simulink model "cube_2d_simulation_model"  (R2015b)
settings: Solver=FixedStepAuto  StartTime=0.0  StopTime=10  FixedStep=T_onboard  RelTol=1e-3
PreLoadFcn:
  | cubeinit
InitFcn:
  | cubeparameters
values from neighbouring files (symbols this model uses):
  a_max = 2*g    [cubeparameters.m]
  a_scaling = 16384    [cubeparameters.m]
  cub_friction = 0.0001    [Linearized_system.m]
  cube_start_angle = 0.1*deg_    (= 0.00174532925199)    [cubeparameters.m]
  deg_ = pi/180    (= 0.0174532925199)    [cubeparameters.m]    (also in testa.m)
  Fcube = 0.0001    [Linearized_system.m]
  Fwheel = 0.05*10^-3    (= 5e-05)    [Linearized_system.m]
  g = 9.81    [CalculateImuErrors2D.m]    (also in Linearized_system.m; plotimudata.m; run_simulation_2D.m)
  I_cube = 2*(I_p + m_s*2*(s/2)^2)      + 2*(I_o + m_s*s^2/4)      + 2*(I_o + m_s*((s/2)^2+s^2))    (= 0.0610225)    [cubeparameters.m]
  I_motor = 1.81*10^-5    (= 1.81e-05)    [Linearized_system.m]
  I_total = 0.035    [Linearized_system.m]
  I_wheel = 8*10^-4    (= 0.0008)    [Linearized_system.m]    (also in cubeparameters.m = 0.000796068)
  imu_intended_alignment = [0;0;-135*deg_]    [cubeparameters.m]
  imu_misalignment = [0;0;0]*deg_    [cubeparameters.m]
  Km_alt = 5.115537e-3    (= 0.005115537)    [cubeparameters.m]
  Kt = 38*10^-3    (= 0.038)    [Linearized_system.m]
  Kv = 36.9*10^-3    (= 0.0369)    [Linearized_system.m]
  L = 0.463*10^-3    (= 0.000463)    [Linearized_system.m]
  l_corner2cog = side_length/sqrt(2)    [cubeparameters.m]
  Lcub = sqrt((mass_centrum_oneside^2)*2) -0.085    [Linearized_system.m]
  Load = 6*10^-4    (= 0.0006)    [Linearized_system.m]
  Lwheel = sqrt((0.1^2)*2) -0.1    [Linearized_system.m]
  mass_cube = 3.487*kg_    (= 3.487)    [cubeparameters.m]    (also in theoreticalmomentofinertia.m)
  maxvinkel = pi/4    (= 0.785398163397)    [Linearized_system.m]
  Mcub = 2.083-Mwheel    (= 1.81)    [Linearized_system.m]
  Mwheel = 0.273    [Linearized_system.m]
  R = 0.608    [Linearized_system.m]    (also in OrientationView.m = (eye(3) - 0.9*A(:, 3)*A(:, 3)'/(A(:, 3)'*A(:, 3))))
  r_cube2imu = e2t([0;0;pi/4])*[55;70;10]*mm_    [cubeparameters.m]
  sensor_seed = 123123    [cubeparameters.m]
  T_onboard = 0.002*s_    (= 0.002)    [cubeparameters.m]
  w_max = 250*deg_/s_    (= 4.36332312999)    [cubeparameters.m]
  w_scaling = 131    [cubeparameters.m]
  wheel_friction = 0.05*10^-3    (= 5e-05)    [Linearized_system.m]
libraries: cube_lib x10, simulink x5, stm32f4_io_lib x2
settings Model: Creator=Stefan  LastModifiedBy=Stefan

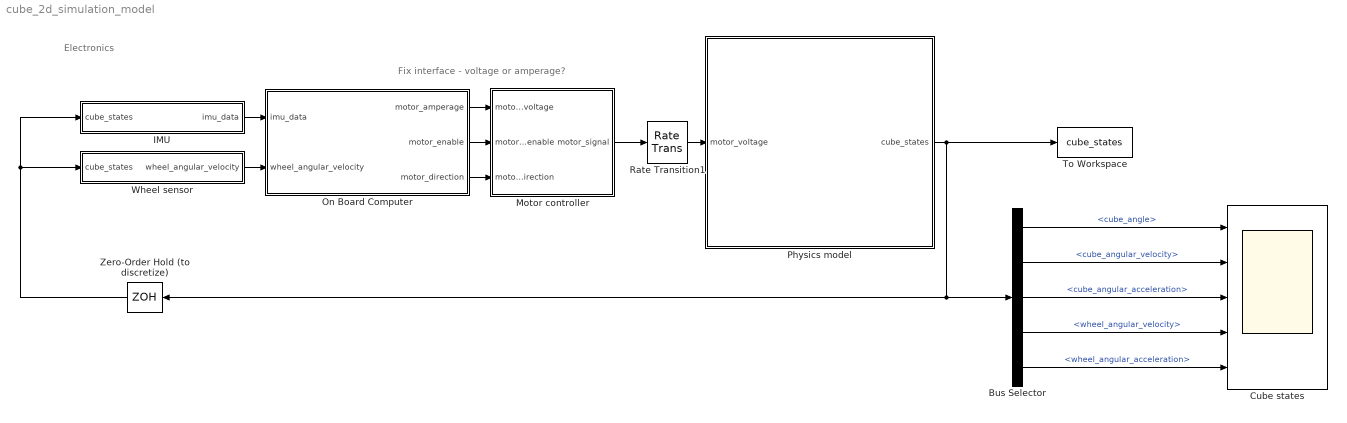
== system cube_2d_simulation_model ==
  note: Fix interface - voltage or amperage?
  note: Electronics
  Bus Selector : BusSelector  OutputSignals=cube_angle,cube_angular_velocity,cube_angular_acceleration,wheel_angular_velocity,wheel_angular_acceleration
  Cube states : Scope  NumInputPorts=5
  IMU : Subsystem
  Motor controller : Subsystem
  On Board Computer : Subsystem
  Physics model : Subsystem
  Rate Transition1 : RateTransition
  To Workspace : ToWorkspace  VariableName=cube_states  SaveFormat=Timeseries  SampleTime=-1
  Wheel sensor : Subsystem
  Zero-Order Hold (to discretize) : ZeroOrderHold  SampleTime=T_onboard
  wires:
  Motor controller/1(motor_signal) -> Rate Transition1/1
  IMU/1(imu_data) -> On Board Computer/1(imu_data)
  On Board Computer/1(motor_amperage) -> Motor controller/1(motor_voltage)
  On Board Computer/2(motor_enable) -> Motor controller/2(motor_enable)
  On Board Computer/3(motor_direction) -> Motor controller/3(motor_direction)
  Wheel sensor/1(wheel_angular_velocity) -> On Board Computer/2(wheel_angular_velocity)
  Zero-Order Hold (to discretize)/1 -> Wheel sensor/1(cube_states), IMU/1(cube_states)
  Rate Transition1/1 -> Physics model/1(motor_voltage)
  Physics model/1(cube_states) -> To Workspace/1, Zero-Order Hold (to discretize)/1, Bus Selector/1
  Bus Selector/2 -> Cube states/2  "<cube_angular_velocity>"
  Bus Selector/4 -> Cube states/4  "<wheel_angular_velocity>"
  Bus Selector/1 -> Cube states/1  "<cube_angle>"
  Bus Selector/3 -> Cube states/3  "<cube_angular_acceleration>"
  Bus Selector/5 -> Cube states/5  "<wheel_angular_acceleration>"

== system cube_2d_simulation_model/IMU ==
  cube_states : Inport
  Add IMU errors : Subsystem
  Convert to IMU output : Subsystem
  To Workspace : ToWorkspace  VariableName=imu_data  SaveFormat=Timeseries  SampleTime=-1
  Transform cube states to IMU states (adds gravity) : MATLAB Function  TreatAsAtomicUnit=on
  imu_data : Outport
  wires:
  cube_states/1 -> Transform cube states to IMU states (adds gravity)/1(cube_states)
  Transform cube states to IMU states (adds gravity)/1(imu_states) -> Add IMU errors/1(true_states)
  Add IMU errors/1(measured_states) -> Convert to IMU output/1(measured_output)
  Convert to IMU output/1(imu_output) -> To Workspace/1, imu_data/1

== system cube_2d_simulation_model/Motor controller ==
  note: Basically, the onboard computer does exactly this but inverted.
      | The conversion and inversion are done to be able to simulate real onboard computer behaviour.
  note: Convert direction to -1/1
  note: 0 (backward) / 1 (forward)
  note: 0/1
  note: Absolute value
  motor_voltage : Inport
  motor_enable : Inport  Port=2
  motor_direction : Inport  Port=3
  Add : Sum
  Constant : Constant  Value=-1
  Gain : Gain  Gain=2
  Product : Product  Inputs=3
  motor_signal : Outport
  wires:
  motor_enable/1 -> Product/2
  motor_voltage/1 -> Product/1
  Product/1 -> motor_signal/1
  Constant/1 -> Add/1
  motor_direction/1 -> Gain/1
  Gain/1 -> Add/2
  Add/1 -> Product/3

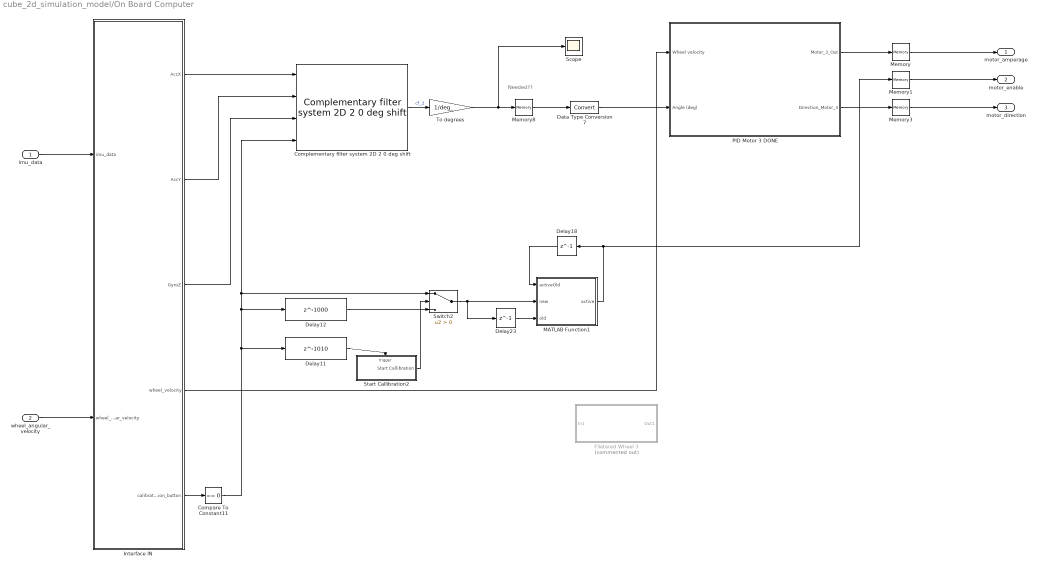
== system cube_2d_simulation_model/On Board Computer ==
  note: Needed??
  imu_data : Inport
  wheel_angular_velocity : Inport  Port=2
  Compare To Constant11 : simulink/Logic and Bit Operations/Compare To Constant  relop===  const=0  OutDataTypeStr=boolean  ZeroCross=off
  Complementary filter system 2D 2 0 deg shift : cube_lib/Complementary filter system 2D 2 0 deg shift
  Data Type Conversion7 : DataTypeConversion
  Delay11 : Delay  DelayLength=1010  InitialCondition=0
  Delay12 : Delay  DelayLength=1000  InitialCondition=0
  Delay18 : Delay  DelayLength=1  InitialCondition=0
  Delay23 : Delay  DelayLength=1  InitialCondition=0
  Filetered Wheel 3 : Subsystem  Commented=on
  Interface IN : Subsystem
  MATLAB Function1 : MATLAB Function  TreatAsAtomicUnit=on
  Memory{,1,3,8} (4 alike) : Memory  InheritSampleTime=on
  "PID Motor 3 DONE " : Subsystem
  Scope : Scope
  Start Callibration2 : Subsystem
  Switch2 : Switch  Criteria=u2 > Threshold
  To degrees : Gain  Gain=1/deg_
  motor_amperage : Outport
  motor_enable : Outport  Port=2
  motor_direction : Outport  Port=3
  wires:
  imu_data/1 -> Interface IN/1(imu_data)
  Data Type Conversion7/1 -> "PID Motor 3 DONE "/2(Angle (deg))
  "PID Motor 3 DONE "/1(Motor_3_Out) -> Memory/1
  Memory8/1 -> Data Type Conversion7/1
  "PID Motor 3 DONE "/2("Direction_Motor_3 ") -> Memory3/1
  Compare To Constant11/1 -> Delay12/1, Complementary filter system 2D 2 0 deg shift/4, Switch2/1, Delay11/1
  MATLAB Function1/1(active) -> Memory1/1, Delay18/1
  Delay23/1 -> MATLAB Function1/3(old)
  Switch2/1 -> Delay23/1, MATLAB Function1/2(new)
  Delay18/1 -> MATLAB Function1/1(activeOld)
  Start Callibration2/1(Start Callibration) -> Switch2/2
  Delay11/1 -> Start Callibration2/Trigger
  Delay12/1 -> Switch2/3
  wheel_angular_velocity/1 -> Interface IN/2(wheel_angular_velocity)
  Memory/1 -> motor_amperage/1
  Memory1/1 -> motor_enable/1
  Memory3/1 -> motor_direction/1
  Interface IN/5(calibration_button) -> Compare To Constant11/1
  Interface IN/4(wheel_velocity) -> "PID Motor 3 DONE "/1(Wheel velocity)
  Interface IN/1(AccX) -> Complementary filter system 2D 2 0 deg shift/1
  Interface IN/2("AccY ") -> Complementary filter system 2D 2 0 deg shift/2
  Interface IN/3(GyroZ) -> Complementary filter system 2D 2 0 deg shift/3
  Complementary filter system 2D 2 0 deg shift/1 -> To degrees/1  "cf_2"
  To degrees/1 -> Scope/1, Memory8/1

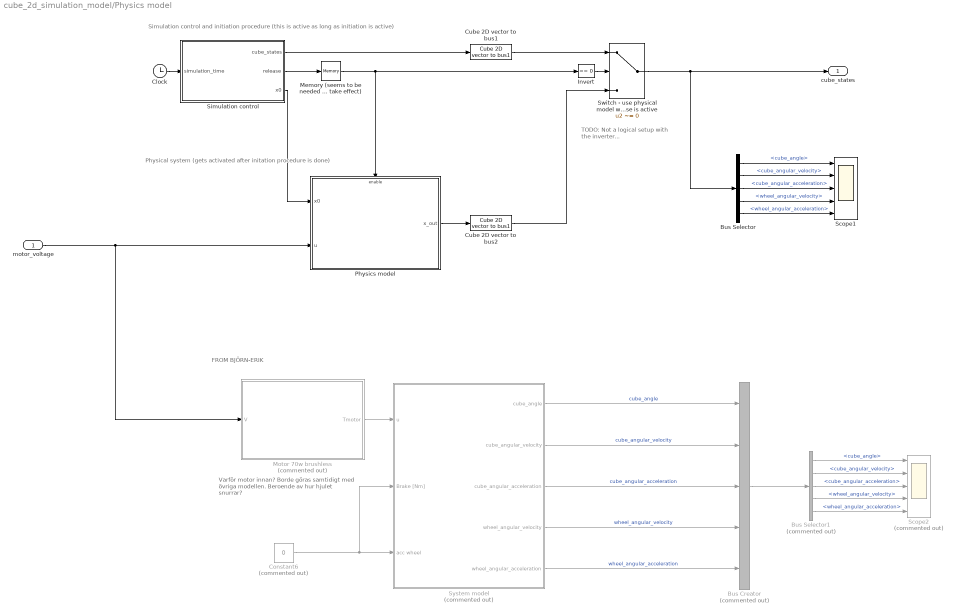
== system cube_2d_simulation_model/Physics model ==
  note: TODO: Not a logical setup
      | with the inverter...
  note: Simulation control and initiation procedure (this is active as long as initiation is active)
  note: Physical system (gets activated after initation procedure is done)
  note: Varför motor innan? Borde göras samtidigt
      | med övriga modellen. Beroende av
      | hur hjulet snurrar?
  note: FROM BJÖRN-ERIK
  motor_voltage : Inport
  Bus Creator : BusCreator  Commented=on  Inputs=5  OutDataTypeStr=Bus: CubeStates2D
  Bus Selector : BusSelector  OutputSignals=cube_angle,cube_angular_velocity,cube_angular_acceleration,wheel_angular_velocity,wheel_angular_acceleration
  Bus Selector1 : BusSelector  Commented=on  OutputSignals=cube_angle,cube_angular_velocity,cube_angular_acceleration,wheel_angular_velocity,wheel_angular_acceleration
  Clock : Clock
  Constant6 : Constant  Commented=on  Value=0
  Cube 2D vector to bus1 : cube_lib/Cube 2D vector to bus1
  Cube 2D vector to bus2 : cube_lib/Cube 2D vector to bus1
  Invert : simulink/Logic and Bit Operations/Compare To Constant  relop===  const=0  OutDataTypeStr=boolean
  Memory (seems to be needed for x0 to take effect) : Memory
  Motor 70w brushless : Subsystem  Commented=on
  Physics model : Subsystem  TreatAsAtomicUnit=on
  Scope1 : Scope  NumInputPorts=5
  Scope2 : Scope  Commented=on  NumInputPorts=5
  Simulation control : MATLAB Function  TreatAsAtomicUnit=on
  Switch - use physical model when release is active : Switch  Criteria=u2 ~= 0
  System model : Subsystem  Commented=on
  cube_states : Outport
  wires:
  System model/2(cube_angular_velocity) -> Bus Creator/2  "cube_angular_velocity"
  System model/3(cube_angular_acceleration) -> Bus Creator/3  "cube_angular_acceleration"
  System model/1(cube_angle) -> Bus Creator/1  "cube_angle"
  System model/4(wheel_angular_velocity) -> Bus Creator/4  "wheel_angular_velocity"
  System model/5(wheel_angular_acceleration) -> Bus Creator/5  "wheel_angular_acceleration"
  Motor 70w brushless/1(Tmotor) -> System model/1(u)
  Constant6/1 -> System model/2(Brake [Nm]), System model/3(acc wheel)
  Bus Selector/2 -> Scope1/2  "<cube_angular_velocity>"
  Bus Selector/1 -> Scope1/1  "<cube_angle>"
  Bus Selector/4 -> Scope1/4  "<wheel_angular_velocity>"
  Bus Selector/5 -> Scope1/5  "<wheel_angular_acceleration>"
  Bus Selector/3 -> Scope1/3  "<cube_angular_acceleration>"
  Cube 2D vector to bus2/1 -> Switch - use physical model when release is active/3
  Bus Selector1/2 -> Scope2/2  "<cube_angular_velocity>"
  Bus Selector1/1 -> Scope2/1  "<cube_angle>"
  Bus Selector1/4 -> Scope2/4  "<wheel_angular_velocity>"
  Bus Selector1/5 -> Scope2/5  "<wheel_angular_acceleration>"
  Bus Selector1/3 -> Scope2/3  "<cube_angular_acceleration>"
  Bus Creator/1 -> Bus Selector1/1
  Clock/1 -> Simulation control/1(simulation_time)
  Simulation control/2(release) -> Memory (seems to be needed for x0 to take effect)/1
  Simulation control/1(cube_states) -> Cube 2D vector to bus1/1
  Cube 2D vector to bus1/1 -> Switch - use physical model when release is active/1
  Switch - use physical model when release is active/1 -> Bus Selector/1, cube_states/1
  Physics model/1(x_out) -> Cube 2D vector to bus2/1
  Simulation control/3(x0) -> Physics model/1(x0)
  Invert/1 -> Switch - use physical model when release is active/2
  Memory (seems to be needed for x0 to take effect)/1 -> Physics model/Enable, Invert/1
  motor_voltage/1 -> Motor 70w brushless/1(V), Physics model/2(u)

== system cube_2d_simulation_model/Wheel sensor ==
  cube_states : Inport
  Bus Selector : BusSelector  OutputSignals=wheel_angular_velocity
  Sensor : cube_lib/Sensor  scale_factor=1  bias=0  noise_std=wheel_noise_standard_deviation  noise_seed=wheel_sensor_seed  sample_time=T_onboard
  wheel_angular_velocity : Outport
  wires:
  Sensor/1 -> wheel_angular_velocity/1
  cube_states/1 -> Bus Selector/1
  Bus Selector/1 -> Sensor/1  "<wheel_angular_velocity>"

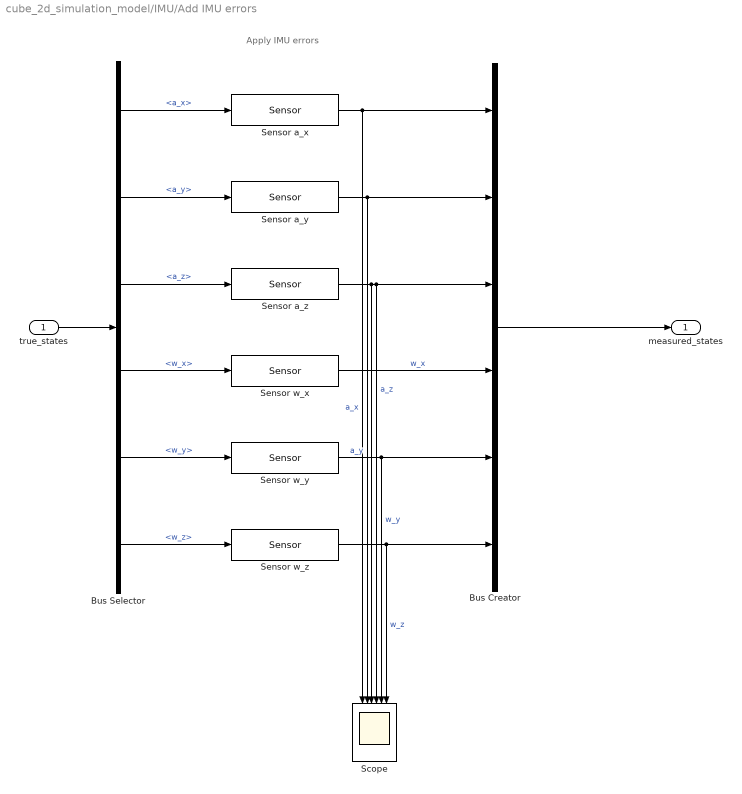
== system cube_2d_simulation_model/IMU/Add IMU errors ==
  note: Apply IMU errors
  true_states : Inport
  Bus Creator : BusCreator  Inputs=6  OutDataTypeStr=Bus: ImuStates
  Bus Selector : BusSelector  OutputSignals=a_x,a_y,a_z,w_x,w_y,w_z
  Scope : Scope  NumInputPorts=6
  Sensor a_x : cube_lib/Sensor  scale_factor=imu_scale_factor_a_x  bias=imu_bias_a_x  noise_std=imu_noise_a_standard_deviation  noise_seed=sensor_seed  sample_time=T_onboard
  Sensor a_y : cube_lib/Sensor  scale_factor=imu_scale_factor_a_y  bias=imu_bias_a_y  noise_std=imu_noise_a_standard_deviation  noise_seed=sensor_seed+1  sample_time=T_onboard
  Sensor a_z : cube_lib/Sensor  scale_factor=imu_scale_factor_a_z  bias=imu_bias_a_z  noise_std=imu_noise_a_standard_deviation  noise_seed=sensor_seed+2  sample_time=T_onboard
  Sensor w_x : cube_lib/Sensor  scale_factor=imu_scale_factor_w_x  bias=imu_bias_w_x  noise_std=imu_noise_w_standard_deviation  noise_seed=sensor_seed+3  sample_time=T_onboard
  Sensor w_y : cube_lib/Sensor  scale_factor=imu_scale_factor_w_y  bias=imu_bias_w_y  noise_std=imu_noise_w_standard_deviation  noise_seed=sensor_seed+4  sample_time=T_onboard
  Sensor w_z : cube_lib/Sensor  scale_factor=imu_scale_factor_w_z  bias=imu_bias_w_z  noise_std=imu_noise_w_standard_deviation  noise_seed=sensor_seed+5  sample_time=T_onboard
  measured_states : Outport
  wires:
  Bus Creator/1 -> measured_states/1
  true_states/1 -> Bus Selector/1
  Bus Selector/6 -> Sensor w_z/1  "<w_z>"
  Sensor a_x/1 -> Scope/1, Bus Creator/1  "a_x"
  Bus Selector/2 -> Sensor a_y/1  "<a_y>"
  Bus Selector/4 -> Sensor w_x/1  "<w_x>"
  Sensor a_y/1 -> Bus Creator/2, Scope/2  "a_y"
  Sensor w_x/1 -> Bus Creator/4  "w_x"
  Sensor w_y/1 -> Bus Creator/5, Scope/5  "w_y"
  Sensor w_z/1 -> Bus Creator/6, Scope/6  "w_z"
  Sensor a_z/1 -> Bus Creator/3, Scope/4, Scope/3  "a_z"
  Bus Selector/5 -> Sensor w_y/1  "<w_y>"
  Bus Selector/3 -> Sensor a_z/1  "<a_z>"
  Bus Selector/1 -> Sensor a_x/1  "<a_x>"

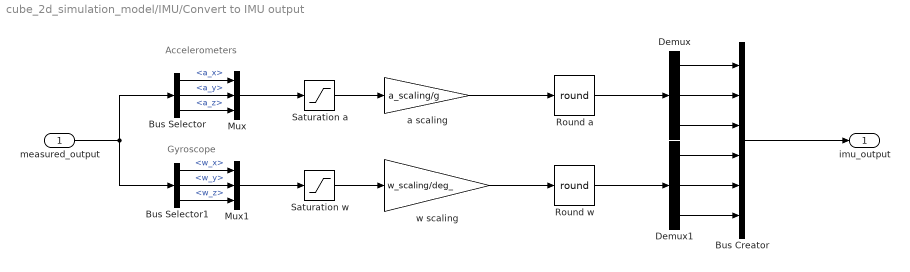
== system cube_2d_simulation_model/IMU/Convert to IMU output ==
  note: Gyroscope
  note: Accelerometers
  measured_output : Inport
  Bus Creator : BusCreator  Inputs=6  OutDataTypeStr=Bus: ImuStates
      settings: InheritFromInputs=off
  Bus Selector : BusSelector  OutputSignals=a_x,a_y,a_z
  Bus Selector1 : BusSelector  OutputSignals=w_x,w_y,w_z
  Demux : Demux  Outputs=3
  Demux1 : Demux  Outputs=3
  Mux : Mux  Inputs=3
  Mux1 : Mux  Inputs=3
  Round a : Rounding  Operator=round
  Round w : Rounding  Operator=round
  Saturation a : Saturate  UpperLimit=a_max  LowerLimit=-a_max
  Saturation w : Saturate  UpperLimit=w_max  LowerLimit=-w_max
  a scaling : Gain  Gain=a_scaling/g
  w scaling : Gain  Gain=w_scaling/deg_
  imu_output : Outport
  wires:
  measured_output/1 -> Bus Selector1/1, Bus Selector/1
  a scaling/1 -> Round a/1
  Saturation a/1 -> a scaling/1
  Saturation w/1 -> w scaling/1
  w scaling/1 -> Round w/1
  Bus Creator/1 -> imu_output/1
  Bus Selector/2 -> Mux/2  "<a_y>"
  Bus Selector/3 -> Mux/3  "<a_z>"
  Bus Selector/1 -> Mux/1  "<a_x>"
  Mux/1 -> Saturation a/1
  Bus Selector1/2 -> Mux1/2  "<w_y>"
  Bus Selector1/3 -> Mux1/3  "<w_z>"
  Bus Selector1/1 -> Mux1/1  "<w_x>"
  Mux1/1 -> Saturation w/1
  Round a/1 -> Demux/1
  Round w/1 -> Demux1/1
  Demux/3 -> Bus Creator/3
  Demux/1 -> Bus Creator/1
  Demux/2 -> Bus Creator/2
  Demux1/3 -> Bus Creator/6
  Demux1/2 -> Bus Creator/5
  Demux1/1 -> Bus Creator/4

== system cube_2d_simulation_model/On Board Computer/Filetered Wheel 3 ==
  In1 : Inport
  Add3 : Sum  Inputs=-+
  Add9 : Sum  Inputs=-+
  Constant1 : Constant  Value=2094  SampleTime=-1
  Constant15 : Constant  Value=69  SampleTime=-1
  Gain2 : Gain  Gain=(6110*2)/4096
  RPM to RAD3 : Gain  Gain=1/9.55
  Scope : Scope
  Out1 : Outport
  wires:
  Gain2/1 -> RPM to RAD3/1
  Add3/1 -> Gain2/1
  Constant1/1 -> Add3/1
  In1/1 -> Add3/2
  Constant15/1 -> Add9/1
  RPM to RAD3/1 -> Add9/2
  Add9/1 -> Scope/1, Out1/1

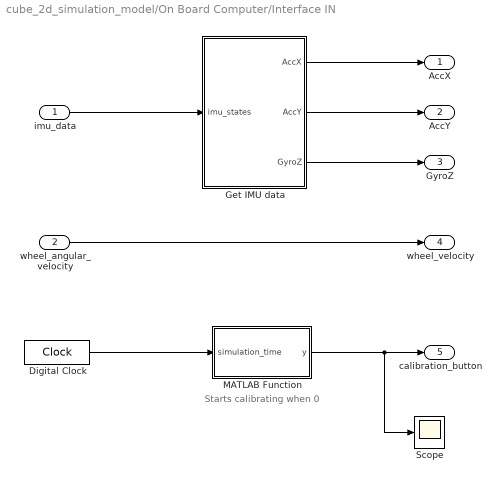
== system cube_2d_simulation_model/On Board Computer/Interface IN ==
  note: Starts calibrating when 0
  imu_data : Inport
  wheel_angular_velocity : Inport  Port=2
  Digital Clock : DigitalClock  SampleTime=T_onboard
  Get IMU data : Subsystem
  MATLAB Function : MATLAB Function  TreatAsAtomicUnit=on
  Scope : Scope
  AccX : Outport
  "AccY " : Outport  Port=2
  GyroZ : Outport  Port=3
  wheel_velocity : Outport  Port=4
  calibration_button : Outport  Port=5
  wires:
  wheel_angular_velocity/1 -> wheel_velocity/1
  imu_data/1 -> Get IMU data/1(imu_states)
  Get IMU data/1(AccX) -> AccX/1
  Get IMU data/2("AccY ") -> "AccY "/1
  Get IMU data/3(GyroZ) -> GyroZ/1
  MATLAB Function/1(y) -> Scope/1, calibration_button/1
  Digital Clock/1 -> MATLAB Function/1(simulation_time)

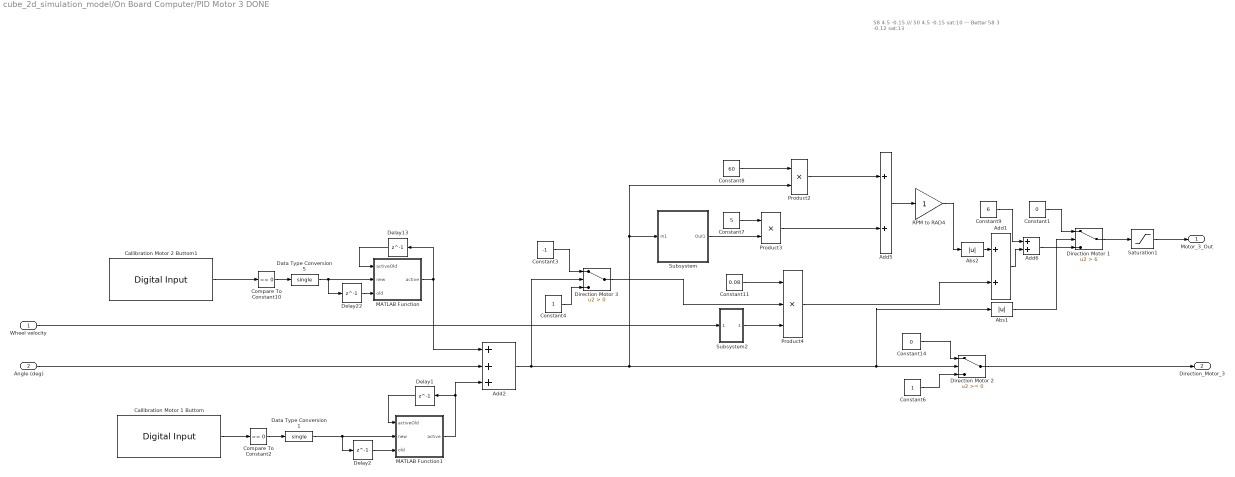
== system cube_2d_simulation_model/On Board Computer/PID Motor 3 DONE  ==
  note: 58
      | 4.5
      | -0.15
      | ///
      | 50
      | 4.5
      | -0.15
      | sat:10
      | --- Better
      | 58
      | 3
      | -0.12
      | sat:13
  Wheel velocity : Inport
  Angle (deg) : Inport  Port=2
  Abs1 : Abs
  Abs2 : Abs
  Add1 : Sum
  Add2 : Sum  Inputs=+++
  Add5 : Sum
  Add6 : Sum
  Callibration Motor 1 Buttom : stm32f4_io_lib/Digital Input  port=E  speed=100  porttype=Pull Up  porttypestr=UP  use_pin0=off  use_pin1=off  use_pin2=off  use_pin3=off  use_pin4=off  use_pin5=off  use_pin6=off  use_pin7=off  use_pin8=off  use_pin9=off  use_pin10=off  use_pin11=off  use_pin12=off  use_pin13=off  use_pin14=on  use_pin15=off  pinstr=GPIO_Pin_14  usedpinarray="[0  0  0  0  0  0  0  0  0  0  0  0  0  0  1  0]"  bitbandingstr="#define OnBoardComputerPIDMotor3DONECallibrationMotor1Buttom_E14 Peripheral_BB(GPIOE->IDR, 14)  /* Output pin */"  sampletime=0.002  sampletimestr=0.002  blockid=OnBoardComputerPIDMotor3DONECallibrationMotor1Buttom  enablecustomportlabel=off  glabalinit=off  cinputportlabel=In1, In2  coutputportlabel=Out1, Out2
  Callibration Motor 2 Buttom1 : stm32f4_io_lib/Digital Input  port=E  speed=100  porttype=Pull Up  porttypestr=UP  use_pin0=off  use_pin1=off  use_pin2=off  use_pin3=off  use_pin4=off  use_pin5=off  use_pin6=off  use_pin7=off  use_pin8=off  use_pin9=off  use_pin10=off  use_pin11=on  use_pin12=off  use_pin13=off  use_pin14=off  use_pin15=off  pinstr=GPIO_Pin_11  usedpinarray="[0  0  0  0  0  0  0  0  0  0  0  1  0  0  0  0]"  bitbandingstr="#define OnBoardComputerPIDMotor3DONECallibrationMotor2Buttom1_E11 Peripheral_BB(GPIOE->IDR, 11)  /* Output pin */"  sampletime=0.002  sampletimestr=0.002  blockid=OnBoardComputerPIDMotor3DONECallibrationMotor2Buttom1  enablecustomportlabel=off  glabalinit=off  cinputportlabel=In1, In2  coutputportlabel=Out1, Out2
  Compare To Constant10 : simulink/Logic and Bit Operations/Compare To Constant  relop===  const=0  OutDataTypeStr=boolean  ZeroCross=off
  Compare To Constant2 : simulink/Logic and Bit Operations/Compare To Constant  relop===  const=0  OutDataTypeStr=boolean  ZeroCross=off
  Constant1 : Constant  Value=0  OutDataTypeStr=single  SampleTime=-1
  Constant11 : Constant  Value=0.08  OutDataTypeStr=single  SampleTime=-1
  Constant14 : Constant  Value=0  OutDataTypeStr=single  SampleTime=-1
  Constant3 : Constant  Value=-1  OutDataTypeStr=single  SampleTime=-1
  Constant4 : Constant  OutDataTypeStr=single  SampleTime=-1
  Constant6 : Constant  OutDataTypeStr=single  SampleTime=-1
  Constant7 : Constant  Value=5  OutDataTypeStr=single  SampleTime=-1
  Constant8 : Constant  Value=60  OutDataTypeStr=single  SampleTime=-1
  Constant9 : Constant  Value=6  SampleTime=-1
  Data Type Conversion1 : DataTypeConversion  OutDataTypeStr=single
  Data Type Conversion5 : DataTypeConversion  OutDataTypeStr=single
  Delay{1..2,13,22} (4 alike) : Delay  DelayLength=1  InitialCondition=0
  Direction Motor 1 : Switch  Criteria=u2 > Threshold  Threshold=6
  Direction Motor 2 : Switch
  Direction Motor 3 : Switch  Criteria=u2 > Threshold
  MATLAB Function : MATLAB Function  TreatAsAtomicUnit=on
  MATLAB Function1 : MATLAB Function  TreatAsAtomicUnit=on
  Product2 : Product
  Product3 : Product
  Product4 : Product  Inputs=3
  RPM to RAD4 : Gain
  Saturation1 : Saturate  UpperLimit=90  LowerLimit=10
  Subsystem : Subsystem
  Subsystem2 : Subsystem
  Motor_3_Out : Outport
  "Direction_Motor_3 " : Outport  Port=2
  wires:
  Direction Motor 2/1 -> "Direction_Motor_3 "/1
  Constant7/1 -> Product3/1
  Constant11/1 -> Product4/1
  Constant14/1 -> Direction Motor 2/1
  Constant6/1 -> Direction Motor 2/3
  Product3/1 -> Add5/2
  Constant9/1 -> Add6/1
  Add5/1 -> RPM to RAD4/1
  RPM to RAD4/1 -> Abs2/1
  Product2/1 -> Add5/1
  Abs2/1 -> Add1/1
  Saturation1/1 -> Motor_3_Out/1
  Constant8/1 -> Product2/1
  Add6/1 -> Direction Motor 1/3
  Direction Motor 1/1 -> Saturation1/1
  Constant1/1 -> Direction Motor 1/1
  Abs1/1 -> Direction Motor 1/2
  Product4/1 -> Add1/2
  Wheel velocity/1 -> Subsystem2/1(In1)
  Angle (deg)/1 -> Add2/2
  Subsystem/1(Out1) -> Product3/2
  Add1/1 -> Add6/2
  Constant4/1 -> Direction Motor 3/3
  Constant3/1 -> Direction Motor 3/1
  Add2/1 -> Direction Motor 3/2, Subsystem/1(In1), Product2/2, Abs1/1, Direction Motor 2/2
  Callibration Motor 2 Buttom1/1 -> Compare To Constant10/1
  Compare To Constant10/1 -> Data Type Conversion5/1
  Callibration Motor 1 Buttom/1 -> Compare To Constant2/1
  Compare To Constant2/1 -> Data Type Conversion1/1
  MATLAB Function/1(active) -> Add2/1, Delay13/1
  Delay22/1 -> MATLAB Function/3(old)
  Data Type Conversion5/1 -> MATLAB Function/2(new), Delay22/1
  Delay13/1 -> MATLAB Function/1(activeOld)
  MATLAB Function1/1(active) -> Add2/3, Delay1/1
  Delay2/1 -> MATLAB Function1/3(old)
  Data Type Conversion1/1 -> Delay2/1, MATLAB Function1/2(new)
  Delay1/1 -> MATLAB Function1/1(activeOld)
  Subsystem2/1(Out2) -> Product4/3
  Direction Motor 3/1 -> Product4/2

== system cube_2d_simulation_model/On Board Computer/Start Callibration2 ==
  Trigger : TriggerPort  PortDimensions=1
  Constant2 : Constant
  Start Callibration : Outport  InitialOutput=[0]
  wires:
  Constant2/1 -> Start Callibration/1

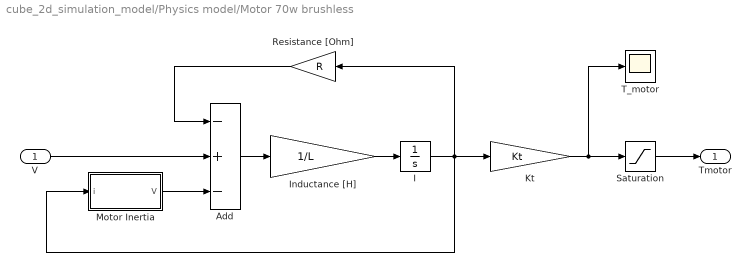
== system cube_2d_simulation_model/Physics model/Motor 70w brushless ==
  V : Inport
  Add : Sum  Inputs=-+-
  I : Integrator
  Inductance [H] : Gain  Gain=1/L
  Kt : Gain  Gain=Kt
  Motor Inertia : Subsystem
  Resistance [Ohm] : Gain  Gain=R
  Saturation : Saturate  UpperLimit=0.128  LowerLimit=-0.128
  T_motor : Scope
  Tmotor : Outport
  wires:
  Add/1 -> Inductance [H]/1
  Resistance [Ohm]/1 -> Add/1
  Inductance [H]/1 -> I/1
  I/1 -> Motor Inertia/1(i), Resistance [Ohm]/1, Kt/1
  Motor Inertia/1(V) -> Add/3
  V/1 -> Add/2
  Kt/1 -> T_motor/1, Saturation/1
  Saturation/1 -> Tmotor/1

== system cube_2d_simulation_model/Physics model/Physics model ==
  x0 : Inport
  u : Inport  Port=2
  Enable : EnablePort
  Create full vector : Subsystem
  Derivative equations : MATLAB Function  TreatAsAtomicUnit=on
  Integrator : Integrator  InitialConditionSource=external  InitialCondition=[cube_start_angle;0;0]
  Scope : Scope
  x_out : Outport
  wires:
  u/1 -> Derivative equations/2(u)
  x0/1 -> Integrator/2
  Derivative equations/1(x_dot) -> Create full vector/2(x_dot), Integrator/1
  Create full vector/1(x_full) -> x_out/1
  Integrator/1 -> Derivative equations/1(x), Scope/1, Create full vector/1(x)

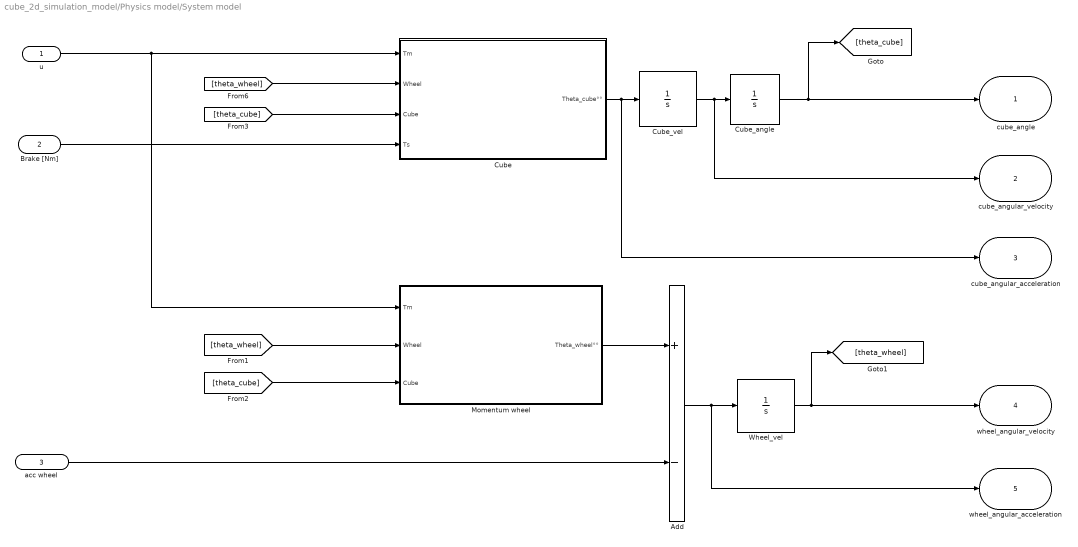
== system cube_2d_simulation_model/Physics model/System model ==
  u : Inport
  Brake [Nm] : Inport  Port=2
  acc wheel : Inport  Port=3
  Add : Sum  Inputs=+-
  Cube : Subsystem
  Cube_angle : Integrator  InitialCondition=cube_start_angle  LimitOutput=on  UpperSaturationLimit=pi/4  LowerSaturationLimit=-pi/4
  Cube_vel : Integrator  UpperSaturationLimit=1  LowerSaturationLimit=0
  Momentum wheel : Subsystem
  Wheel_vel : Integrator  LimitOutput=on  UpperSaturationLimit=4800/9.55  LowerSaturationLimit=-4800/9.55
  cube_angle : Outport
  cube_angular_velocity : Outport  Port=2
  cube_angular_acceleration : Outport  Port=3
  wheel_angular_velocity : Outport  Port=4
  wheel_angular_acceleration : Outport  Port=5
  wires:
  Cube_angle/1 -> [theta_cube], cube_angle/1
  Cube_vel/1 -> cube_angular_velocity/1, Cube_angle/1
  Momentum wheel/1(Theta_wheel°°) -> Add/1
  Cube/1(Theta_cube°°) -> cube_angular_acceleration/1, Cube_vel/1
  [theta_cube] -> Cube/3(Cube)
  [theta_wheel] -> Cube/2(Wheel)
  [theta_wheel] -> Momentum wheel/2(Wheel)
  [theta_cube] -> Momentum wheel/3(Cube)
  Wheel_vel/1 -> [theta_wheel], wheel_angular_velocity/1
  u/1 -> Momentum wheel/1(Tm), Cube/1(Tm)
  Add/1 -> wheel_angular_acceleration/1, Wheel_vel/1
  acc wheel/1 -> Add/2
  Brake [Nm]/1 -> Cube/4(Ts)

== system cube_2d_simulation_model/On Board Computer/Interface IN/Get IMU data ==
  imu_states : Inport
  Bus Selector : BusSelector  OutputSignals=a_x,a_y,w_z
  AccX : Outport
  "AccY " : Outport  Port=2
  GyroZ : Outport  Port=3
  wires:
  imu_states/1 -> Bus Selector/1
  Bus Selector/1 -> AccX/1  "<a_x>"
  Bus Selector/2 -> "AccY "/1  "<a_y>"
  Bus Selector/3 -> GyroZ/1  "<w_z>"

== system cube_2d_simulation_model/On Board Computer/PID Motor 3 DONE /Subsystem ==
  In1 : Inport
  DUMMY7 : Terminator
  Discrete Derivative : simulink/Discrete/Discrete Derivative  gainval=1.0  ICPrevScaledInput=0.0  InputProcessing=Inherited  OutMin=[]  OutMax=[]  OutDataType=fixdt(1, 16)  OutScaling=2^-10  DoSatur=off
  Do average zero2 : If  NumInputs=2  IfExpression=u1 == u2
  Subsystem2 : Subsystem
  Unit Delay1 : UnitDelay  SampleTime=-1
  Out1 : Outport
  wires:
  Do average zero2/2 -> Subsystem2/Action
  Unit Delay1/1 -> Do average zero2/2
  Discrete Derivative/1 -> Out1/1  "Cube angle velocity [degree/s]"
  Subsystem2/1(Out1) -> Discrete Derivative/1
  In1/1 -> Subsystem2/1(In1), Unit Delay1/1, Do average zero2/1
  Do average zero2/1 -> DUMMY7/1

== system cube_2d_simulation_model/On Board Computer/PID Motor 3 DONE /Subsystem2 ==
  In1 : Inport
  DUMMY7 : Terminator
  Do average zero1 : If  NumInputs=2  IfExpression=u1 == u2
  Subsystem1 : Subsystem
  Unit Delay3 : UnitDelay  SampleTime=-1
  Out2 : Outport
  wires:
  Unit Delay3/1 -> Do average zero1/2
  Do average zero1/2 -> Subsystem1/Action
  In1/1 -> Subsystem1/1(In1), Unit Delay3/1, Do average zero1/1
  Subsystem1/1(Out1) -> Out2/1
  Do average zero1/1 -> DUMMY7/1

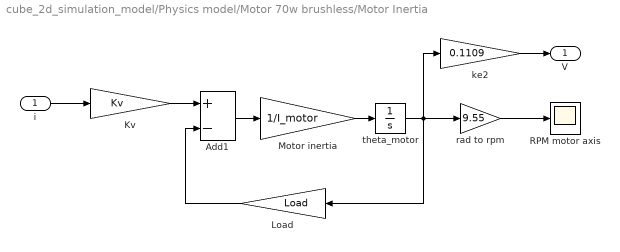
== system cube_2d_simulation_model/Physics model/Motor 70w brushless/Motor Inertia ==
  i : Inport
  Add1 : Sum  Inputs=+-
  Kv : Gain  Gain=Kv
  Load : Gain  Gain=Load
  Motor inertia : Gain  Gain=1/I_motor
  "RPM motor axis " : Scope
  ke2 : Gain  Gain=0.1109
  rad to rpm : Gain  Gain=9.55
  theta_motor : Integrator
  V : Outport
  wires:
  theta_motor/1 -> Load/1, ke2/1, rad to rpm/1
  Motor inertia/1 -> theta_motor/1
  Add1/1 -> Motor inertia/1
  Kv/1 -> Add1/1
  i/1 -> Kv/1
  ke2/1 -> V/1
  Load/1 -> Add1/2
  rad to rpm/1 -> "RPM motor axis "/1

== system cube_2d_simulation_model/Physics model/Physics model/Create full vector ==
  x : Inport
  x_dot : Inport  Port=2
  Demux : Demux  Outputs=3
  Demux1 : Demux  Outputs=3
  Mux : Mux  Inputs=5
  Terminator1 : Terminator
  x_full : Outport
  wires:
  Demux/3 -> Mux/4  "wheel_angular_velocity"
  Demux1/3 -> Mux/5  "wheel_angular_acceleration"
  Mux/1 -> x_full/1
  Demux1/2 -> Mux/3  "cube_angular_acceleration"
  Demux/2 -> Mux/2  "cube_angular_velocity"
  Demux/1 -> Mux/1  "cube_angle"
  Demux1/1 -> Terminator1/1
  x/1 -> Demux/1
  x_dot/1 -> Demux1/1

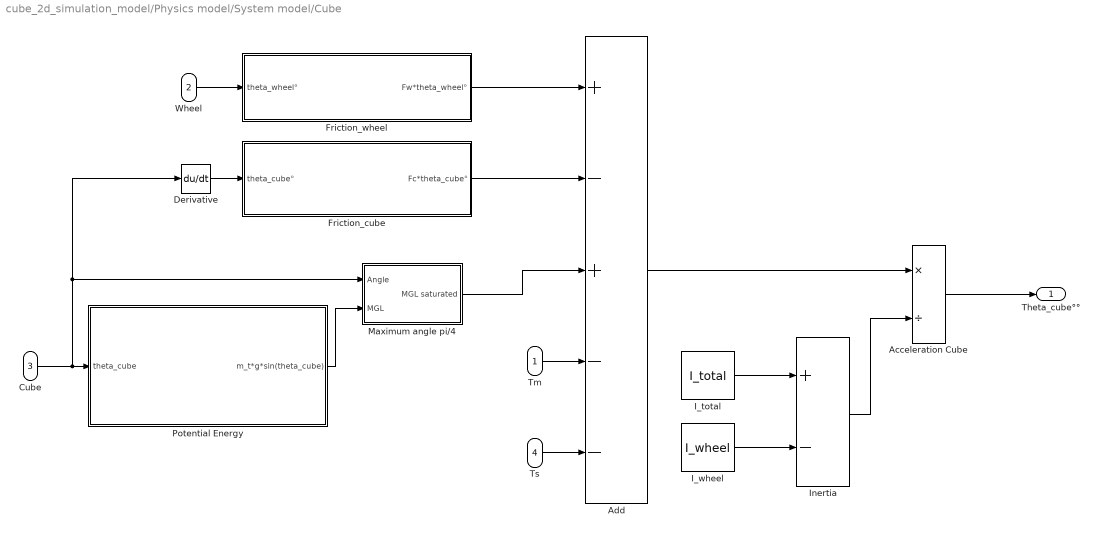
== system cube_2d_simulation_model/Physics model/System model/Cube ==
  Tm : Inport
  Wheel : Inport  Port=2
  Cube : Inport  Port=3
  Ts : Inport  Port=4
  Acceleration Cube : Product  Inputs=*/
  Add : Sum  Inputs=+-+--
  Derivative : Derivative
  Friction_cube : Subsystem
  Friction_wheel : Subsystem
  I_total : Constant  Value=I_total
  I_wheel : Constant  Value=I_wheel
  Inertia : Sum  Inputs=+-
  "Maximum angle pi/4 " : Subsystem
  Potential Energy : Subsystem
  Theta_cube°° : Outport
  wires:
  Inertia/1 -> Acceleration Cube/2
  I_total/1 -> Inertia/1
  Acceleration Cube/1 -> Theta_cube°°/1
  I_wheel/1 -> Inertia/2
  Friction_cube/1(Fc*theta_cube°) -> Add/2
  Friction_wheel/1(Fw*theta_wheel°) -> Add/1
  Wheel/1 -> Friction_wheel/1(theta_wheel°)
  Derivative/1 -> Friction_cube/1(theta_cube°)
  Ts/1 -> Add/5
  Add/1 -> Acceleration Cube/1
  Cube/1 -> Derivative/1, "Maximum angle pi/4 "/1("Angle "), Potential Energy/1(theta_cube)
  "Maximum angle pi/4 "/1("MGL saturated ") -> Add/3
  Tm/1 -> Add/4
  Potential Energy/1(m_t*g*sin(theta_cube)) -> "Maximum angle pi/4 "/2(MGL)

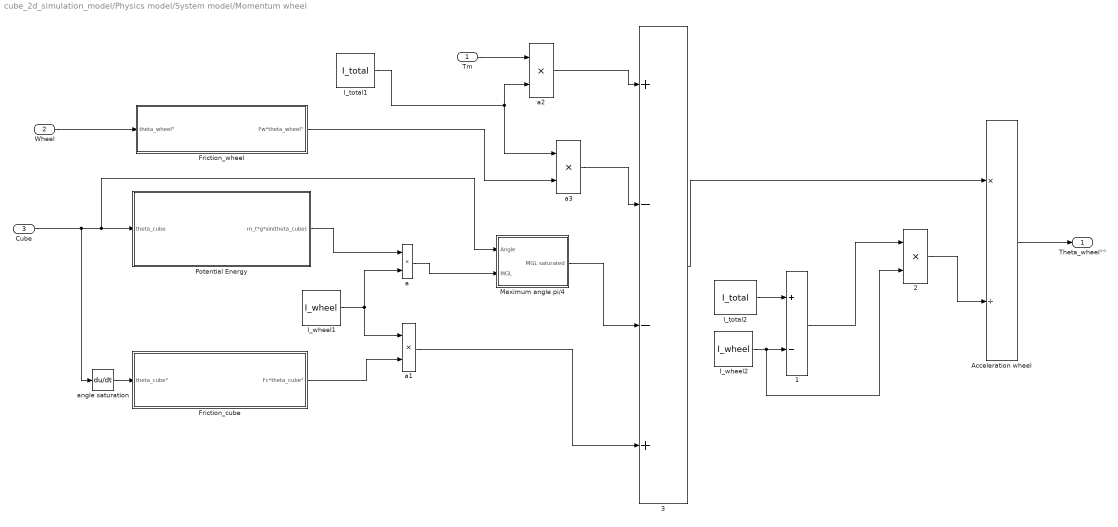
== system cube_2d_simulation_model/Physics model/System model/Momentum wheel ==
  Tm : Inport
  Wheel : Inport  Port=2
  Cube : Inport  Port=3
  1 : Sum  Inputs=+-
  2 : Product  Inputs=**
  3 : Sum  Inputs=+--+
  Acceleration wheel : Product  Inputs=*/
  Friction_cube : Subsystem
  Friction_wheel : Subsystem
  I_total1 : Constant  Value=I_total
  I_total2 : Constant  Value=I_total
  I_wheel1 : Constant  Value=I_wheel
  I_wheel2 : Constant  Value=I_wheel
  Maximum angle pi/4 : Subsystem
  Potential Energy : Subsystem
  a{,1..3} (4 alike) : Product  Inputs=**
  angle saturation : Derivative
  Theta_wheel°° : Outport
  wires:
  2/1 -> Acceleration wheel/2
  I_total2/1 -> 1/1
  Friction_cube/1(Fc*theta_cube°) -> a1/2
  a3/1 -> 3/2
  I_wheel2/1 -> 2/2, 1/2
  Acceleration wheel/1 -> Theta_wheel°°/1
  Potential Energy/1(m_t*g*sin(theta_cube)) -> a/1
  a2/1 -> 3/1
  1/1 -> 2/1
  Friction_wheel/1(Fw*theta_wheel°) -> a3/2
  Tm/1 -> a2/1
  a1/1 -> 3/4
  I_total1/1 -> a2/2, a3/1
  I_wheel1/1 -> a/2, a1/1
  Wheel/1 -> Friction_wheel/1(theta_wheel°)
  angle saturation/1 -> Friction_cube/1(theta_cube°)
  3/1 -> Acceleration wheel/1
  Cube/1 -> Maximum angle pi/4/1("Angle "), Potential Energy/1(theta_cube), angle saturation/1
  a/1 -> Maximum angle pi/4/2(MGL)
  Maximum angle pi/4/1("MGL saturated ") -> 3/3

== system cube_2d_simulation_model/On Board Computer/PID Motor 3 DONE /Subsystem/Subsystem2 ==
  In1 : Inport
  Action Port : ActionPort  ActionType=else
  Subsystem : Subsystem
  Unit Delay1 : UnitDelay  SampleTime=-1
  Out1 : Outport
  wires:
  In1/1 -> Subsystem/1(In1)
  Subsystem/1(Average Speed) -> Out1/1  "Speed, PA1"
  Subsystem/2(One old Speed) -> Unit Delay1/1
  Unit Delay1/1 -> Subsystem/2(One old speed)

== system cube_2d_simulation_model/On Board Computer/PID Motor 3 DONE /Subsystem2/Subsystem1 ==
  In1 : Inport
  Action Port : ActionPort  ActionType=else
  Subsystem : Subsystem
  Unit Delay1 : UnitDelay  SampleTime=-1
  Out1 : Outport
  wires:
  In1/1 -> Subsystem/1(In1)
  Subsystem/1(Average Speed) -> Out1/1  "Speed, PA1"
  Subsystem/2(One old Speed) -> Unit Delay1/1
  Unit Delay1/1 -> Subsystem/2(One old speed)

== system cube_2d_simulation_model/Physics model/System model/Cube/Friction_cube ==
  theta_cube° : Inport
  Friction Cube vs Floor : Constant  Value=cub_friction
  Product : Product
  Fc*theta_cube° : Outport
  wires:
  Friction Cube vs Floor/1 -> Product/1
  Product/1 -> Fc*theta_cube°/1
  theta_cube°/1 -> Product/2

== system cube_2d_simulation_model/Physics model/System model/Cube/Friction_wheel ==
  theta_wheel° : Inport
  Friction wheel : Constant  Value=wheel_friction
  Product : Product
  Fw*theta_wheel° : Outport
  wires:
  theta_wheel°/1 -> Product/2
  Product/1 -> Fw*theta_wheel°/1
  Friction wheel/1 -> Product/1

== system cube_2d_simulation_model/Physics model/System model/Cube/Maximum angle pi//4  ==
  "Angle " : Inport
  MGL : Inport  Port=2
  MATLAB Function : MATLAB Function  TreatAsAtomicUnit=on
  maximum angle the cube can have i.e when lying at the floor +-45° : Constant  Value=maxvinkel
  "MGL saturated " : Outport
  wires:
  MGL/1 -> MATLAB Function/3(value)
  MATLAB Function/1(y) -> "MGL saturated "/1
  "Angle "/1 -> MATLAB Function/2(angle)
  maximum angle the cube can have i.e when lying at the floor +-45°/1 -> MATLAB Function/1(maxvinkelConst)

== system cube_2d_simulation_model/Physics model/System model/Cube/Potential Energy ==
  theta_cube : Inport
  "Gravitation acceleration " : Constant  Value=g
  MATLAB Function : MATLAB Function  TreatAsAtomicUnit=on
  Mass times the length of wheel and cube : Subsystem
  Product2 : Product  Inputs=3
  m_t*g*sin(theta_cube) : Outport
  wires:
  Product2/1 -> m_t*g*sin(theta_cube)/1
  theta_cube/1 -> MATLAB Function/1(u)
  MATLAB Function/1(y) -> Product2/1
  "Gravitation acceleration "/1 -> Product2/2
  Mass times the length of wheel and cube/1(Ltmt) -> Product2/3

== system cube_2d_simulation_model/Physics model/System model/Momentum wheel/Friction_cube ==
  theta_cube° : Inport
  Constant9 : Constant  Value=cub_friction
  Product : Product
  Fc*theta_cube° : Outport
  wires:
  Constant9/1 -> Product/1
  Product/1 -> Fc*theta_cube°/1
  theta_cube°/1 -> Product/2

== system cube_2d_simulation_model/Physics model/System model/Momentum wheel/Friction_wheel ==
  theta_wheel° : Inport
  Constant2 : Constant  Value=wheel_friction
  Product : Product
  Fw*theta_wheel° : Outport
  wires:
  theta_wheel°/1 -> Product/2
  Product/1 -> Fw*theta_wheel°/1
  Constant2/1 -> Product/1

== system cube_2d_simulation_model/Physics model/System model/Momentum wheel/Maximum angle pi//4 ==
  "Angle " : Inport
  MGL : Inport  Port=2
  MATLAB Function : MATLAB Function  TreatAsAtomicUnit=on
  maximum angle when cube lying at the floor +- 45° : Constant  Value=maxvinkel
  "MGL saturated " : Outport
  wires:
  MGL/1 -> MATLAB Function/3(value)
  MATLAB Function/1(y) -> "MGL saturated "/1
  "Angle "/1 -> MATLAB Function/2(angle)
  maximum angle when cube lying at the floor +- 45°/1 -> MATLAB Function/1(maxvinkelConst)

== system cube_2d_simulation_model/Physics model/System model/Momentum wheel/Potential Energy ==
  theta_cube : Inport
  Constant3 : Constant  Value=g
  Ltmt : Subsystem
  MATLAB Function : MATLAB Function  TreatAsAtomicUnit=on
  Product2 : Product  Inputs=3
  m_t*g*sin(theta_cube) : Outport
  wires:
  Product2/1 -> m_t*g*sin(theta_cube)/1
  theta_cube/1 -> MATLAB Function/1(u)
  MATLAB Function/1(y) -> Product2/1
  Constant3/1 -> Product2/2
  Ltmt/1(Ltmt) -> Product2/3

== system cube_2d_simulation_model/On Board Computer/PID Motor 3 DONE /Subsystem/Subsystem2/Subsystem ==
  In1 : Inport
  One old speed : Inport  Port=2
  Add2 : Sum
  Gain2 : Gain  Gain=0.5
  Gain3 : Gain  Gain=0.5
  Average Speed : Outport
  One old Speed : Outport  Port=2
  wires:
  Add2/1 -> One old Speed/1, Average Speed/1  "Speed, PA1"
  One old speed/1 -> Gain2/1
  In1/1 -> Gain3/1
  Gain2/1 -> Add2/2
  Gain3/1 -> Add2/1

== system cube_2d_simulation_model/On Board Computer/PID Motor 3 DONE /Subsystem2/Subsystem1/Subsystem ==
  In1 : Inport
  One old speed : Inport  Port=2
  Add2 : Sum
  Gain2 : Gain  Gain=0.3
  Gain3 : Gain  Gain=0.7
  Average Speed : Outport
  One old Speed : Outport  Port=2
  wires:
  Add2/1 -> One old Speed/1, Average Speed/1  "Speed, PA1"
  One old speed/1 -> Gain2/1
  In1/1 -> Gain3/1
  Gain2/1 -> Add2/2
  Gain3/1 -> Add2/1

== system cube_2d_simulation_model/Physics model/System model/Cube/Potential Energy/Mass times the length of wheel and cube ==
  Add : Sum
  Constant : Constant  Value=Mcub
  Constant1 : Constant  Value=Mwheel
  Constant4 : Constant  Value=Lcub
  Constant6 : Constant  Value=Lwheel
  Product : Product
  Product1 : Product
  Ltmt : Outport
  wires:
  Constant/1 -> Product/1
  Add/1 -> Ltmt/1
  Constant1/1 -> Product1/1
  Constant6/1 -> Product1/2
  Product/1 -> Add/1
  Constant4/1 -> Product/2
  Product1/1 -> Add/2

== system cube_2d_simulation_model/Physics model/System model/Momentum wheel/Potential Energy/Ltmt ==
  Add : Sum
  Constant : Constant  Value=Mcub
  Constant1 : Constant  Value=Mwheel
  Constant4 : Constant  Value=Lcub
  Constant6 : Constant  Value=Lwheel
  Product : Product
  Product1 : Product
  Ltmt : Outport
  wires:
  Constant1/1 -> Product1/1
  Constant4/1 -> Product/2
  Product/1 -> Add/1
  Constant/1 -> Product/1
  Add/1 -> Ltmt/1
  Constant6/1 -> Product1/2
  Product1/1 -> Add/2

== matlab function cube_2d_simulation_model/On Board Computer/PID Motor 3 DONE /MATLAB Function ==
  data: activeOld input; active output; new input; old input
function active  = fcn(activeOld,new,old)
    if(new == 1 && old == 0)
        active = activeOld+0.05;
    else
        active = activeOld;
    end
end

== matlab function cube_2d_simulation_model/IMU/Transform cube states to IMU states (adds gravity) ==
  data: cube_states input Bus: CubeStates2D; imu_states output Bus: ImuStates; r_cube2imu parameter; imu_intended_alignment parameter; imu_misalignment parameter
function imu_states = CubeToImuStates(cube_states, r_cube2imu,imu_intended_alignment,imu_misalignment)
%#codegen
% Converts cube states to IMU states by changing reference frame
g = 9.82; 

persistent C_b_s; % Does not change

if isempty(C_b_s)
    C_b_s = e2t(-imu_intended_alignment-imu_misalignment); % Body to sensor. Verifiera tecken
end

% Read data
cube_angle                  = cube_states.cube_angle;
cube_angular_velocity       = cube_states.cube_angular_velocity;
cube_angular_acceleration   = cube_states.cube_angular_acceleration;

w = [0;0;cube_angular_velocity];
w_dot = [0;0;cube_angular_acceleration];
r_vec = e2t([0;0;cube_angle])*r_cube2imu;
g_vec = g*[0;1;0];

% Transformation matrices
C_i_b = e2t([0;0;-cube_angle]); % Inertial to body. Verifiera tecken

% Body reference frame, inertial coordinates
w_imu_i = [0;0;cube_angular_velocity];
a_imu_i = cross(w_dot,r_vec) + cross(w,cross(w,r_vec)) + g_vec;

% Body reference frame, sensor coordinates
w_imu_s = w_imu_i; % Rotating around the same axis
a_imu_s = C_b_s*C_i_b*a_imu_i;

% Copy to output and scale according to data sheet
imu_states.a_x = a_imu_s(1);
imu_states.a_y = a_imu_s(2);
imu_states.a_z = a_imu_s(3);

imu_states.w_x = w_imu_s(1);
imu_states.w_y = w_imu_s(2);
imu_states.w_z = w_imu_s(3);

== matlab function cube_2d_simulation_model/On Board Computer/PID Motor 3 DONE /MATLAB Function1 ==
  data: activeOld input; active output; new input; old input
function active  = fcn(activeOld,new,old)
    if(new == 1 && old == 0)
        active = activeOld-0.05;
    else
        active = activeOld;
    end
end

== matlab function cube_2d_simulation_model/Physics model/Physics model/Derivative equations ==
  data: x input; u input; x_dot output double; Fcube parameter; Fwheel parameter; mass_cube parameter; I_cube parameter; I_wheel parameter; l_corner2cog parameter; Km_alt parameter
function x_dot = CubeDerivative2D(x,u,Fcube,Fwheel,mass_cube,I_cube,I_wheel,l_corner2cog,Km_alt)
%#codegen
% x and x_dot are vectors
%
% States:
% cube_angle
% cube_angular_velocity
% wheel_angular_velocity
% Negative cube angle is when MOTOR 3 text on cube is horizontal

% To shorten variable names, the following aliases are used
% _w: Wheel
% _c: Cube
% _f: f
% w:  Angular velocity
% a:  Angular acceleration
% th: Angle

% Read values
g       = 9.82;
th_c    = x(1); % cube angle
w_c     = x(2); % cube angular velocity
w_w     = x(3); % wheel angular velocity
F_c     = Fcube;
F_w     = Fwheel;
m_t     = mass_cube;
I_f     = I_cube;
I_w     = I_wheel;
L_t     = l_corner2cog;
K_m     = Km_alt;

% Calculate derivatives
% Using T_motor = Km*u
a_c = (L_t*m_t*g*sin(th_c) - K_m*u + F_w*w_w - F_c*w_c)/I_f;
a_w = (K_m*u*(I_f + I_w) - F_w*w_w*(I_f + I_w) - L_t*m_t*g*sin(th_c)*I_w + F_c*w_c*I_w)/(I_f*I_w);

% Write values
x_dot = [
    w_c     % d/dt(cube_angle)
    a_c     % d/dt(cube_angular_velocity)
    a_w     % d/dt(wheel_angular_velocity)(
    ];

== matlab function cube_2d_simulation_model/Physics model/System model/Cube/Maximum angle pi//4 /MATLAB Function ==
  data: maxvinkelConst input; angle input; y output; value input
function y = fcn(maxvinkelConst,angle, value)
%#codegens

if angle >= maxvinkelConst 
    y=0;
elseif angle <= -maxvinkelConst
    y =0;
else
    y = value;
end

== matlab function cube_2d_simulation_model/Physics model/System model/Cube/Potential Energy/MATLAB Function ==
  data: u input; y output
function y = fcn(u)
%#codegen

y = sin(u);

== matlab function cube_2d_simulation_model/Physics model/System model/Momentum wheel/Maximum angle pi//4/MATLAB Function ==
  data: maxvinkelConst input; angle input; y output; value input
function y = fcn(maxvinkelConst,angle, value)
%#codegens

if angle >= maxvinkelConst 
    y=0;
elseif angle <= -maxvinkelConst
    y =0;
else
    y = value;
end

== matlab function cube_2d_simulation_model/Physics model/System model/Momentum wheel/Potential Energy/MATLAB Function ==
  data: u input; y output
function y = fcn(u)
%#codegen

%y= -2*cos(u-pi/4)*sin(u-pi/4)
%y = -2*sin(2*u);
y = sin(u);

== matlab function cube_2d_simulation_model/Physics model/Simulation control ==
  data: cube_states output; release output; x0 output; simulation_time input; cube_start_angle parameter
function [cube_states,release,x0] = SimulationControl(simulation_time,cube_start_angle)
%#codegen
% Here the initiation procedure can be programmed. 
% Current procedure: The cube lies on one side for a number of seconds
% to let the navigation algorithm find errors. Then it is placed close to
% the balancing angle and released.

deg_ = pi/180;
s_ = 1;

% type, start_time, start_angle
% time: starting time of the current pose
% angle: angle of cube
% release: if 1, the cube is allowed to move according to the physics
%          if 0, it is controlled by this procedure
% Procedure gives velocity continuous transfer between angles
% Last procedure angle gives release
procedure = [
    0*s_,   -45*deg_
    2.5*s_, -45*deg_
    3.5*s_, 45*deg_
    6*s_,   45*deg_
    7*s_,   cube_start_angle
    ];

% Read data
% Find current procedure row. Use temporary variable r_temp to convince 
% Simulink compiler that r is scalar.
r_temp = find(procedure(:,1) <= simulation_time,1,'last');
if isempty(r_temp)
    r = 1;
    disp('Warning: no valid procedure.')
else
    r = r_temp(1); % To ensure scalarity
end

if r == size(procedure,1) % last row
    release = 1;
    cube_angle = procedure(r,2);
    cube_angular_velocity = 0;
else
    release = 0;
    start_angle = procedure(r,2);
    stop_angle  = procedure(r+1,2);
    start_time  = procedure(r,1);
    stop_time   = procedure(r+1,1);

    cube_angular_velocity = (stop_angle-start_angle)/(stop_time-start_time);

    cube_angle = start_angle+(simulation_time-start_time)*cube_angular_velocity;
end

% Write data
cube_states = [cube_angle;cube_angular_velocity;0;0;0];

if release
    x0 = [procedure(r,2);0;0];
else
    x0 = zeros(3,1);
end

== matlab function cube_2d_simulation_model/On Board Computer/Interface IN/MATLAB Function ==
  data: simulation_time input; y output
function y = Calibration(simulation_time)
%#codegen

if simulation_time == 0
    y = 1;
elseif simulation_time > 0 && simulation_time < 0.1
    y = 0;
elseif simulation_time > 3.5 && simulation_time < 3.7
    y = 0;
else
    y = 1;
end

== matlab function cube_2d_simulation_model/On Board Computer/MATLAB Function1 ==
  data: activeOld input; active output; new input; old input
function active  = fcn(activeOld,new,old)
    if(new == 1 && old == 0)
        if(activeOld ==0)
            active = 1;
        else 
            active = 0;
        end 
    else
        active = activeOld;
    end
end
